simulink model "mpc_rf_boiler"  (R2017a)
settings: Solver=FixedStepAuto  StartTime=0.0  StopTime=simTime  FixedStep=Dt  RelTol=1e-3  EnableMultiTasking=on
values from neighbouring files (symbols this model uses):
  beta = [0.0001 0.0001 0.0001]    [mpc_design_parameters_0706.mat]
  bFilter = 1    [mpcBoiler_0206.m]
  controlClosedLoop = 1    [mpcBoiler_0206.m]
  D0 = 35.7834    [mpc_design_parameters_0706.mat]    (also in mpc_fixed_parameters_0706.mat)
  Dt = 1    [mpcBoiler_0206.m]
  GAParameters = [200 50 37 1e-06 3 10 1 0 1e-06 10 9]    [mpc_design_parameters_0706.mat]
  lambdaMatrix = [0.0001 0.0001 0.0001 0.0001 0.0001 0.0001 0.0001 0.0001 0.0001 0.0001 0.0001 0.0001 ... (30 elements, 3x10)]    [mpc_design_parameters_0706.mat]
  lBounds = [-5 -5 -5 -5 -5 -5 -5 -5 -5]    [mpc_design_parameters_0706.mat]
  maxDDelay = 2    [mpc_design_parameters_0706.mat]    (also in mpc_fixed_parameters_0706.mat)
  maxUDelay = 2    [mpc_design_parameters_0706.mat]    (also in mpc_fixed_parameters_0706.mat)
  maxYDelay = 4    [mpc_design_parameters_0706.mat]    (also in mpc_fixed_parameters_0706.mat)
  na = [4 4 4]    [mpc_design_parameters_0706.mat]    (also in mpc_fixed_parameters_0706.mat)
  nb = [1  1  1; 2  2  2; 2  2  2]    [mpc_design_parameters_0706.mat]    (also in mpc_fixed_parameters_0706.mat)
  nc = [1 2 2]    [mpc_design_parameters_0706.mat]    (also in mpc_fixed_parameters_0706.mat)
  nPredictors = [8 12 12]    [mpc_design_parameters_0706.mat]    (also in mpc_fixed_parameters_0706.mat)
  nTrees = [100 100 100]    [mpc_design_parameters_0706.mat]    (also in mpc_fixed_parameters_0706.mat)
  qMatrix = [1e-05 1 1 1e-05 1 1 1e-05 1 1 1e-05 1 1 ... (27 elements, 3x9)]    [mpc_design_parameters_0706.mat]
  rMatrix = [1  1  1; 1  1  1; 0.01  0.01  0.01]    [mpc_design_parameters_0706.mat]
  tau_C = 12*tau_R    (= 60)    [mpcBoiler_0206.m]
  tau_R = 5    [mpcBoiler_0206.m]
  U0 = [32.9816 46.2282 25.3416]    [mpc_design_parameters_0706.mat]    (also in mpc_fixed_parameters_0706.mat)
  uBounds = [5 5 5 5 5 5 5 5 5]    [mpc_design_parameters_0706.mat]
  uLims = [0 0 0 0 0 0 0 0 0 100 100 100 ... (18 elements, 3x3x2)]    [mpc_design_parameters_0706.mat]
  Y0 = [41.412 28.7553 38.6037]    [mpc_design_parameters_0706.mat]    (also in mpc_fixed_parameters_0706.mat)
  yLims = [0 27.317535 0 0 27.317535 0 0 27.317535 0 0 27.317535 0 ... (60 elements, 3x10x2)]    [mpc_design_parameters_0706.mat]
settings Model: Creator=Pablo Diaz  LastModifiedBy=Pablo Diaz
settings OptimizationCC: LifeSpan=inf
settings DebuggingCC: SFUnexpectedBacktrackingDiag=warning  SFNoUnconditionalDefaultTransitionDiag=warning  SFExecutionAtInitializationDiag=none
settings GRTTargetCC: TargetLangStandard=C89/C90 (ANSI)
settings ConfigComp: CovMetricSettings=dw  CovHtmlReporting=on  CovSaveCumulativeToWorkspaceVar=on  CovSaveSingleToWorkspaceVar=on  CovExternalEMLEnable=off

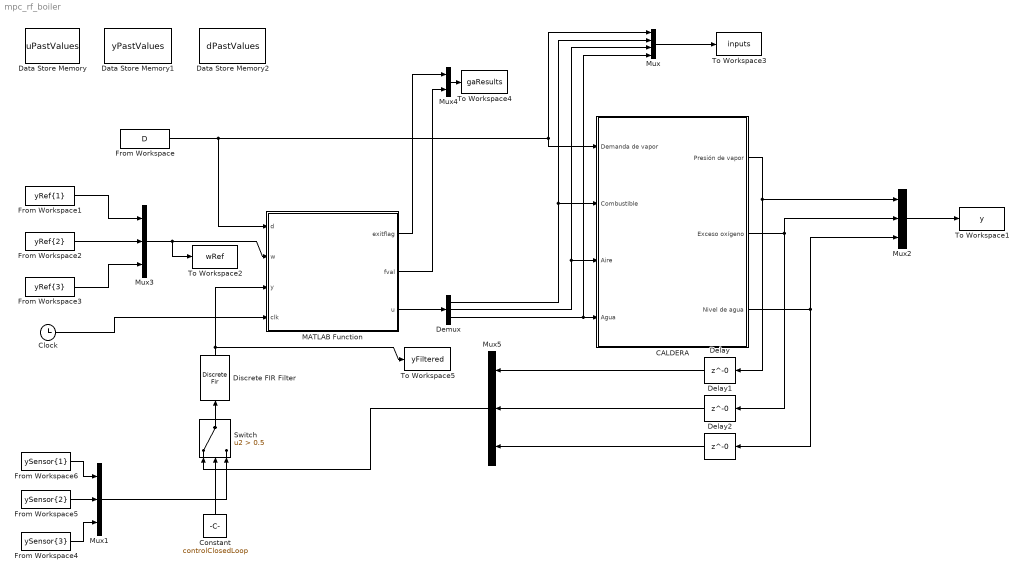
== system mpc_rf_boiler ==
  CALDERA : Subsystem
  Clock : Clock
  Constant : Constant  Value=controlClosedLoop
  Data Store Memory : DataStoreMemory  DataStoreName=uPastValues  ReadBeforeWriteMsg=warning  WriteAfterWriteMsg=warning  WriteAfterReadMsg=warning  InitialValue=[U0]'*ones(1,maxUDelay);  VectorParams1D=off  ShowAdditionalParam=off  OutDataTypeStr=double
  Data Store Memory1 : DataStoreMemory  DataStoreName=yPastValues  ReadBeforeWriteMsg=warning  WriteAfterWriteMsg=warning  WriteAfterReadMsg=warning  InitialValue=Y0'*ones(1,maxYDelay)  VectorParams1D=off  ShowAdditionalParam=off  OutDataTypeStr=double
  Data Store Memory2 : DataStoreMemory  DataStoreName=dPastValues  ReadBeforeWriteMsg=warning  WriteAfterWriteMsg=warning  WriteAfterReadMsg=warning  InitialValue=D0'*ones(1,maxDDelay)  VectorParams1D=off  ShowAdditionalParam=off  OutDataTypeStr=double
  Delay : Delay  DelayLength=0  InitialCondition=Y0(1)
  Delay1 : Delay  DelayLength=0  InitialCondition=Y0(2)
  Delay2 : Delay  DelayLength=0  InitialCondition=Y0(3)
  Demux : Demux  Outputs=3
  Discrete FIR Filter : DiscreteFir  Coefficients=bFilter
  From Workspace : FromWorkspace  VariableName=D  SampleTime=Dt  Interpolate=off  OutputAfterFinalValue=Holding final value
  From Workspace1 : FromWorkspace  VariableName=yRef{1}  SampleTime=Dt  Interpolate=off  OutputAfterFinalValue=Holding final value
  From Workspace2 : FromWorkspace  VariableName=yRef{2}  SampleTime=0  Interpolate=off  OutputAfterFinalValue=Holding final value
  From Workspace3 : FromWorkspace  VariableName=yRef{3}  SampleTime=Dt  Interpolate=off  OutputAfterFinalValue=Holding final value
  From Workspace4 : FromWorkspace  VariableName=ySensor{3}  SampleTime=Dt  Interpolate=off  OutputAfterFinalValue=Holding final value
  From Workspace5 : FromWorkspace  VariableName=ySensor{2}  SampleTime=Dt  Interpolate=off  OutputAfterFinalValue=Holding final value
  From Workspace6 : FromWorkspace  VariableName=ySensor{1}  SampleTime=Dt  Interpolate=off  OutputAfterFinalValue=Holding final value
  MATLAB Function : MATLAB Function  TreatAsAtomicUnit=on
  Mux : Mux
  Mux{1..3,5} (4 alike) : Mux  Inputs=3
  Mux4 : Mux  Inputs=2
  Switch : Switch  Criteria=u2 > Threshold  Threshold=0.5
  To Workspace1 : ToWorkspace  VariableName=y  SaveFormat=Structure With Time  SampleTime=-1
  To Workspace2 : ToWorkspace  VariableName=wRef  SaveFormat=Structure With Time  SampleTime=-1
  To Workspace3 : ToWorkspace  VariableName=inputs  SaveFormat=Structure With Time  SampleTime=-1
  To Workspace4 : ToWorkspace  VariableName=gaResults  SaveFormat=Structure With Time  SampleTime=-1
  To Workspace5 : ToWorkspace  VariableName=yFiltered  SaveFormat=Structure With Time  SampleTime=-1
  wires:
  Mux/1 -> To Workspace3/1
  MATLAB Function/3(u) -> Demux/1
  Mux3/1 -> To Workspace2/1, MATLAB Function/2(w)
  From Workspace1/1 -> Mux3/1
  From Workspace2/1 -> Mux3/2
  From Workspace3/1 -> Mux3/3
  MATLAB Function/1(exitflag) -> Mux4/1
  Mux4/1 -> To Workspace4/1
  MATLAB Function/2(fval) -> Mux4/2
  Clock/1 -> MATLAB Function/4(clk)
  Discrete FIR Filter/1 -> To Workspace5/1, MATLAB Function/3(y)
  From Workspace5/1 -> Mux1/2
  From Workspace6/1 -> Mux1/1
  From Workspace4/1 -> Mux1/3
  Delay/1 -> Mux5/1
  Delay1/1 -> Mux5/2
  Delay2/1 -> Mux5/3
  Demux/3 -> Mux/4, CALDERA/4(Agua)
  CALDERA/2(Exceso oxígeno) -> Mux2/2, Delay1/1
  Mux2/1 -> To Workspace1/1
  CALDERA/3(Nivel de agua) -> Mux2/3, Delay2/1
  Demux/2 -> Mux/3, CALDERA/3(Aire)
  From Workspace/1 -> MATLAB Function/1(d), Mux/1, CALDERA/1(Demanda de vapor)
  Demux/1 -> Mux/2, CALDERA/2(Combustible)
  CALDERA/1(Presión de vapor) -> Delay/1, Mux2/1
  Switch/1 -> Discrete FIR Filter/1
  Constant/1 -> Switch/2
  Mux5/1 -> Switch/1
  Mux1/1 -> Switch/3

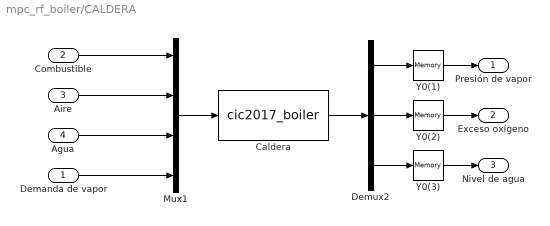
== system mpc_rf_boiler/CALDERA ==
  Demanda de vapor : Inport
  Combustible : Inport  Port=2
  Aire : Inport  Port=3
  Agua : Inport  Port=4
  Caldera : S-Function  FunctionName=cic2017_boiler  Parameters=Y0,[U0 D0]  SFunctionDeploymentMode=off  EnableBusSupport=off
  Demux2 : Demux  Outputs=3
  Mux1 : Mux
  Y0(1) : Memory  X0=Y0(1)
  Y0(2) : Memory  X0=Y0(2)
  Y0(3) : Memory  X0=Y0(3)
  Presión de vapor : Outport
  Exceso oxígeno : Outport  Port=2
  Nivel de agua : Outport  Port=3
  wires:
  Caldera/1 -> Demux2/1
  Aire/1 -> Mux1/2
  Agua/1 -> Mux1/3
  Demanda de vapor/1 -> Mux1/4
  Combustible/1 -> Mux1/1
  Mux1/1 -> Caldera/1
  Demux2/1 -> Y0(1)/1
  Demux2/2 -> Y0(2)/1
  Demux2/3 -> Y0(3)/1
  Y0(1)/1 -> Presión de vapor/1
  Y0(2)/1 -> Exceso oxígeno/1
  Y0(3)/1 -> Nivel de agua/1

== matlab function mpc_rf_boiler/MATLAB Function ==
  data: exitflag output; fval output; d input; w input; y input; clk input; u output; qMatrix parameter; rMatrix parameter; lambdaMatrix parameter; beta parameter; yLims parameter; lBounds parameter; uBounds parameter; nTrees parameter; nPredictors parameter; na parameter; nb parameter; nc parameter; yPastValues data_store_memory; uPastValues data_store_memory; dPastValues data_store_memory; tau_R parameter; tau_C parameter; uLims parameter; GAParameters parameter
function [exitflag, fval, u] = MPC_RF(d, w, y, clk,...
                                    qMatrix, rMatrix, lambdaMatrix, beta,...
                                    yLims, lBounds, uBounds, ...
                                    nTrees, nPredictors, na, nb, nc,...
                                    tau_R, tau_C,...
                                    uLims,GAParameters)
coder.extrinsic('mpc_wrapper_ga');
global yPastValues
global uPastValues
global dPastValues
[m,N_u] = size(rMatrix);
nPopulation = GAParameters(1);
%% Extrinsic pre declaration
UNow = [0 0 0]';
fval = NaN;
exitflag = NaN;
population = zeros(nPopulation,m*N_u); % Change after
scores = zeros(nPopulation,1);
%%
if rem(clk,tau_R) == 0
    % Sample time for tau_R has been hit
    
    % Refresh past sequences of Y and D with new measured value
    yPastValues(:,2:end) = yPastValues(:,1:(end-1));
    dPastValues(:,2:end) = dPastValues(:,1:(end-1));
    yPastValues(:,1) = y;
    dPastValues(:,1) = d;
    if rem(clk,tau_C) == 0
        % Compute optimal MV values (saturated inside)
        wMatrix = mpc_generate_w_matrix(w,qMatrix);
        [UNow,fval,exitflag,population,scores] = mpc_wrapper_ga(yPastValues,uPastValues,dPastValues,...
                                                              qMatrix,rMatrix,lambdaMatrix,beta,wMatrix,...
                                                              yLims,uLims,lBounds,uBounds,...
                                                              nTrees,nPredictors,na,nb,nc,...
                                                              GAParameters);
    else
        % Keep MV in past values if no MPC computation was required
        UNow = uPastValues(:,1);
    end
    uPastValues(:,2:end) = uPastValues(:,1:(end-1));
    uPastValues(:,1) = UNow;
else
    % Keep MV in past values if not
    UNow = uPastValues(:,1);
end
u = UNow;
